simulink model "que5_3"  (R2023a)
settings: Solver=VariableStepAuto  StartTime=0.0  StopTime=100  RelTol=1e-3
values from neighbouring files (symbols this model uses):
  A = [0 1 0 0 ... (first row only)    [que5_1.m]    (also in que5_1_1.m; que5_4.m; que6_1.m = [0 1 0; que6_2_sim_input.m = [0 1 0;0 0 1;0 0 -0.5])
  B = [0 ... (first row only)    [que5_1.m]    (also in que5_1_1.m; que5_4.m; que6_1.m = [0 0 0.5]'; que6_2_sim_input.m = [0;0;0.5])
  C = [1,0, 0, 0 ... (first row only)    [que5_1.m]    (also in que5_1_1.m; que5_4.m = [1, 0, 0, 0]; que6_1.m = [1 0 0; que6_2_sim_input.m = [1 0 0)
settings Model: Creator=Hasee  LastModifiedBy=Administrator

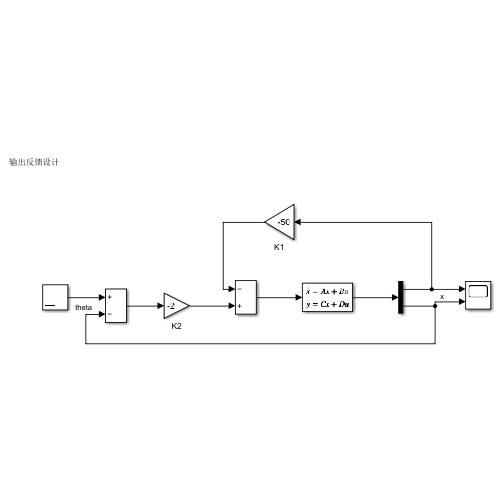
[thumbnail: Simulink's stored preview of the top-level diagram]
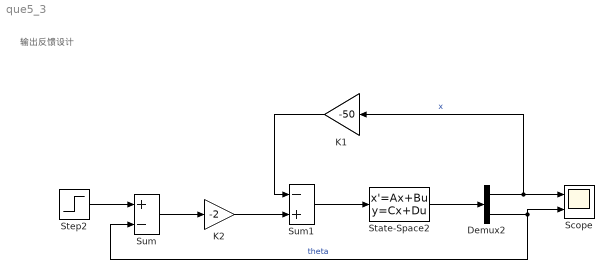
== system que5_3 ==
  note: 输出反馈设计
  Demux2 : Demux  Outputs=2
  K1 : Gain  Gain=-50
  K2 : Gain  Gain=-2
  Scope : Scope  NumInputPorts=2
  State-Space2 : StateSpace  A=A  B=B  C=C  D=[0 0]'  InitialCondition=0
  Step2 : Step  Time=5  SampleTime=0
  Sum : Sum  Inputs=+-
  Sum1 : Sum  Inputs=-+
  wires:
  Sum/1 -> K2/1
  Step2/1 -> Sum/1
  K2/1 -> Sum1/2
  K1/1 -> Sum1/1
  Sum1/1 -> State-Space2/1
  State-Space2/1 -> Demux2/1
  Demux2/1 -> K1/1, Scope/1  "x"
  Demux2/2 -> Sum/2, Scope/2  "theta"
